simulink model "gm_UZ_EnDat_be4_segregation"  (R2023b)
settings: Solver=FixedStepAuto  StartTime=0  StopTime=0.000505  RelTol=1e-3
model workspace (MAT data in the model file):
  Select = 0
libraries: hdlsllib x74, simulink x21, hdlmdlgenlib x4, simulink_extras x1
(part 5 of 5)

== system gm_UZ_EnDat_be4_segregation/UZ_ENDAT/ManualDeserializere/ramwatcher/Increment Stored Integer ==
  u : Inport  OutDataTypeStr=fixdt(0,16,0,'DataTypeOverride', 'Off')  SampleTime=1e-08
  FixPt Constant : Constant  DisableCoverage=on  OutDataTypeStr=Inherit: Inherit via back propagation  SampleTime=-1
  FixPt Data Type Duplicate : DataTypeDuplicate  DisableCoverage=on  NumInputPorts=3
  FixPt Gateway In : DataTypeConversion  DisableCoverage=on  ConvertRealWorld=Stored Integer (SI)  SaturateOnIntegerOverflow=off  RndMeth=Floor
  FixPt Sum1 : Sum  OutDataTypeStr=Inherit: Inherit via back propagation  InputSameDT=on  LockScale=on
  sigspec : SignalSpecification  OutDataTypeStr=uint16  Dimensions=1
  y : Outport  SampleTime=1e-08  InitialOutput=0
  wires:
  u/1 -> FixPt Sum1/1, FixPt Data Type Duplicate/2
  FixPt Constant/1 -> sigspec/1
  FixPt Gateway In/1 -> FixPt Sum1/2, FixPt Data Type Duplicate/3
  FixPt Sum1/1 -> FixPt Data Type Duplicate/1, y/1
  sigspec/1 -> FixPt Gateway In/1

== system gm_UZ_EnDat_be4_segregation/UZ_ENDAT/ManualSerialize/CLKCNTER_RECIEVE/Positional_Counter ==
  valueout : Inport  OutDataTypeStr=uint32  PortDimensions=1  SampleTime=1e-08
  Trigger : Inport  Port=2  OutDataTypeStr=boolean  SampleTime=1e-08
  Increment Stored Integer : Subsystem  mask(Stored Integer Value Increment){}
      mask help: Simulink:masks:StoredIntegerValueIncrement_MD
      mask Display: disp('Q++')
  Increment Stored Integer_out1bypassMux : MultiPortSwitch  DataPortOrder=Zero-based contiguous  Inputs=2  zeroidx=on  OutDataTypeStr=uint32  SampleTime=1e-08  SaturateOnIntegerOverflow=off  InputSameDT=off
  Trigger_delay : Delay  DelayLength=double(1)  InitialCondition=0
  Trigger_delayed_inverted_and_Trigger : Logic  AllPortsSameDT=off  OutDataTypeStr=boolean  SampleTime=1e-08
  not_Trigger_delayed : Logic  Operator=NOT  Inputs=1  AllPortsSameDT=off  OutDataTypeStr=boolean  SampleTime=1e-08
  out0_bypass : UnitDelay  InitialCondition="fi(0,0,32,0,\"hex\",\"00000000\")"  SampleTime=1e-08
  divider : Outport  SampleTime=1e-08  InitialOutput=0
  wires:
  Trigger/1 -> Trigger_delayed_inverted_and_Trigger/2, Trigger_delay/1
  valueout/1 -> Increment Stored Integer/1(u)
  Increment Stored Integer_out1bypassMux/1 -> divider/1, out0_bypass/1
  Trigger_delay/1 -> not_Trigger_delayed/1
  not_Trigger_delayed/1 -> Trigger_delayed_inverted_and_Trigger/1
  Trigger_delayed_inverted_and_Trigger/1 -> Increment Stored Integer_out1bypassMux/1
  out0_bypass/1 -> Increment Stored Integer_out1bypassMux/2
  Increment Stored Integer/1(y) -> Increment Stored Integer_out1bypassMux/3

== system gm_UZ_EnDat_be4_segregation/UZ_ENDAT/ManualSerialize/CLKCNTER_RECIEVE/SetZero32 ==
  valin : Inport  OutDataTypeStr=uint32  PortDimensions=1  SampleTime=1e-08
  setzero : Inport  Port=2  OutDataTypeStr=boolean  PortDimensions=1  SampleTime=1e-08
  Trigger : Inport  Port=3  OutDataTypeStr=boolean  SampleTime=1e-08
  Constant1 : Constant  OutDataTypeStr=fixdt(0, 1, 0)  SampleTime=1e-08
  Constant2 : Constant  Value=0  OutDataTypeStr=fixdt(0, 1, 0)  SampleTime=1e-08
  Index Vector1 : MultiPortSwitch  DataPortOrder=Zero-based contiguous  Inputs=2  DiagnosticForDefault=None  zeroidx=on  OutDataTypeStr=fixdt(0, 1, 0)  SampleTime=1e-08  SaturateOnIntegerOverflow=off  InputSameDT=off
  Product : Product  Inputs=**  OutDataTypeStr=uint32  SaturateOnIntegerOverflow=on  SampleTime=1e-08
  Product_out1bypassMux : MultiPortSwitch  DataPortOrder=Zero-based contiguous  Inputs=2  zeroidx=on  OutDataTypeStr=uint32  SampleTime=1e-08  SaturateOnIntegerOverflow=off  InputSameDT=off
  Trigger_delay : Delay  DelayLength=double(1)  InitialCondition=0
  Trigger_delay_Initial_Val : Constant  OutDataTypeStr=boolean  SampleTime=1e-08
  Trigger_delay_ctrl_const : Constant  OutDataTypeStr=boolean  SampleTime=1e-08
  Trigger_delay_ctrl_delay : Delay  DelayLength=double(1)  InitialCondition=0
  Trigger_delay_switch : Switch  Criteria=u2 ~= 0  Threshold=double(0)  OutDataTypeStr=boolean  SampleTime=1e-08  SaturateOnIntegerOverflow=off  InputSameDT=off
  Trigger_delayed_inverted_and_Trigger : Logic  AllPortsSameDT=off  OutDataTypeStr=boolean  SampleTime=1e-08
  delayMatch{,1..5} (6 alike) : Delay  DelayLength=double(2)  InitialCondition=0
  not_Trigger_delayed : Logic  Operator=NOT  Inputs=1  AllPortsSameDT=off  OutDataTypeStr=boolean  SampleTime=1e-08
  out0_bypass : UnitDelay  InitialCondition=double(0)  SampleTime=1e-08
  out0_bypass_Initial_Val : Constant  OutDataTypeStr=uint32  SampleTime=1e-08
  out0_bypass_ctrl_const : Constant  OutDataTypeStr=boolean  SampleTime=1e-08
  out0_bypass_ctrl_delay : Delay  DelayLength=double(1)  InitialCondition=0
  out0_bypass_switch : Switch  Criteria=u2 ~= 0  Threshold=double(0)  OutDataTypeStr=uint32  SampleTime=1e-08  SaturateOnIntegerOverflow=off  InputSameDT=off
  valueout : Outport  SampleTime=1e-08  InitialOutput=0  VectorParamsAs1DForOutWhenUnconnected=off
  wires:
  Trigger/1 -> Trigger_delayed_inverted_and_Trigger/2, Trigger_delay/1
  valin/1 -> Product/2
  setzero/1 -> Index Vector1/1
  Trigger_delay_switch/1 -> not_Trigger_delayed/1
  not_Trigger_delayed/1 -> Trigger_delayed_inverted_and_Trigger/1
  Trigger_delay/1 -> Trigger_delay_switch/1
  delayMatch1/1 -> Trigger_delay_switch/3
  delayMatch/1 -> Trigger_delay_switch/2
  Index Vector1/1 -> Product/1
  delayMatch2/1 -> Index Vector1/2
  delayMatch3/1 -> Index Vector1/3
  Trigger_delay_ctrl_delay/1 -> delayMatch/1
  Trigger_delay_Initial_Val/1 -> delayMatch1/1
  Constant1/1 -> delayMatch2/1
  Constant2/1 -> delayMatch3/1
  out0_bypass_ctrl_delay/1 -> delayMatch4/1
  out0_bypass_Initial_Val/1 -> delayMatch5/1
  Product_out1bypassMux/1 -> out0_bypass/1, valueout/1
  out0_bypass/1 -> out0_bypass_switch/1
  delayMatch4/1 -> out0_bypass_switch/2
  delayMatch5/1 -> out0_bypass_switch/3
  Trigger_delayed_inverted_and_Trigger/1 -> Product_out1bypassMux/1
  Product/1 -> Product_out1bypassMux/3
  out0_bypass_switch/1 -> Product_out1bypassMux/2
  out0_bypass_ctrl_const/1 -> out0_bypass_ctrl_delay/1
  Trigger_delay_ctrl_const/1 -> Trigger_delay_ctrl_delay/1

== system gm_UZ_EnDat_be4_segregation/UZ_ENDAT/ManualSerialize/Storage16/Compare To Zero ==
  u : Inport  OutDataTypeStr=fixdt(0,64,0,'DataTypeOverride', 'Off')  SampleTime=1e-08
  Compare : RelationalOperator  Operator===  OutDataTypeStr=boolean
  Constant : Constant  DisableCoverage=on  Value=0  OutDataTypeStr=Inherit: Inherit via back propagation  SampleTime=-1  PreserveConstantTs=on
  y : Outport  SampleTime=1e-08
  wires:
  u/1 -> Compare/1
  Compare/1 -> y/1
  Constant/1 -> Compare/2

== system gm_UZ_EnDat_be4_segregation/UZ_ENDAT/Subsystem/CLKCNTERBOOTUP/Positional_Counter ==
  valueout : Inport  OutDataTypeStr=fixdt(0, 64, 0)  PortDimensions=1  SampleTime=1e-08
  Trigger : Inport  Port=2  OutDataTypeStr=boolean  SampleTime=1e-08
  Increment Stored Integer : Subsystem  mask(Stored Integer Value Increment){}
      mask help: Simulink:masks:StoredIntegerValueIncrement_MD
      mask Display: disp('Q++')
  Increment Stored Integer_out1bypassMux : MultiPortSwitch  DataPortOrder=Zero-based contiguous  Inputs=2  zeroidx=on  OutDataTypeStr=fixdt(0, 64, 0)  SampleTime=1e-08  SaturateOnIntegerOverflow=off  InputSameDT=off
  Trigger_delay : Delay  DelayLength=double(1)  InitialCondition=0
  Trigger_delayed_inverted_and_Trigger : Logic  AllPortsSameDT=off  OutDataTypeStr=boolean  SampleTime=1e-08
  not_Trigger_delayed : Logic  Operator=NOT  Inputs=1  AllPortsSameDT=off  OutDataTypeStr=boolean  SampleTime=1e-08
  out0_bypass : UnitDelay  InitialCondition="fi(0,0,64,0,\"hex\",\"0000000000000000\")"  SampleTime=1e-08
  divider : Outport  SampleTime=1e-08  InitialOutput=0
  wires:
  Trigger/1 -> Trigger_delayed_inverted_and_Trigger/2, Trigger_delay/1
  valueout/1 -> Increment Stored Integer/1(u)
  Increment Stored Integer_out1bypassMux/1 -> divider/1, out0_bypass/1
  Trigger_delay/1 -> not_Trigger_delayed/1
  not_Trigger_delayed/1 -> Trigger_delayed_inverted_and_Trigger/1
  Trigger_delayed_inverted_and_Trigger/1 -> Increment Stored Integer_out1bypassMux/1
  out0_bypass/1 -> Increment Stored Integer_out1bypassMux/2
  Increment Stored Integer/1(y) -> Increment Stored Integer_out1bypassMux/3

== system gm_UZ_EnDat_be4_segregation/UZ_ENDAT/Subsystem/CLKCNTERBOOTUP/SetZero64 ==
  valin : Inport  OutDataTypeStr=fixdt(0, 64, 0)  PortDimensions=1  SampleTime=1e-08
  setzero : Inport  Port=2  OutDataTypeStr=boolean  PortDimensions=1  SampleTime=1e-08
  Trigger : Inport  Port=3  OutDataTypeStr=boolean  SampleTime=1e-08
  Constant1 : Constant  OutDataTypeStr=fixdt(0, 1, 0)  SampleTime=1e-08
  Constant2 : Constant  Value=0  OutDataTypeStr=fixdt(0, 1, 0)  SampleTime=1e-08
  Index Vector1 : MultiPortSwitch  DataPortOrder=Zero-based contiguous  Inputs=2  DiagnosticForDefault=None  zeroidx=on  OutDataTypeStr=fixdt(0, 1, 0)  SampleTime=1e-08  SaturateOnIntegerOverflow=off  InputSameDT=off
  Product : Product  Inputs=**  OutDataTypeStr=fixdt(0, 64, 0)  SaturateOnIntegerOverflow=on  SampleTime=1e-08
  Product_out1bypassMux : MultiPortSwitch  DataPortOrder=Zero-based contiguous  Inputs=2  zeroidx=on  OutDataTypeStr=fixdt(0, 64, 0)  SampleTime=1e-08  SaturateOnIntegerOverflow=off  InputSameDT=off
  Trigger_delay : Delay  DelayLength=double(1)  InitialCondition=0
  Trigger_delay_Initial_Val : Constant  OutDataTypeStr=boolean  SampleTime=1e-08
  Trigger_delay_ctrl_const : Constant  OutDataTypeStr=boolean  SampleTime=1e-08
  Trigger_delay_ctrl_delay : Delay  DelayLength=double(1)  InitialCondition=0
  Trigger_delay_switch : Switch  Criteria=u2 ~= 0  Threshold=double(0)  OutDataTypeStr=boolean  SampleTime=1e-08  SaturateOnIntegerOverflow=off  InputSameDT=off
  Trigger_delayed_inverted_and_Trigger : Logic  AllPortsSameDT=off  OutDataTypeStr=boolean  SampleTime=1e-08
  not_Trigger_delayed : Logic  Operator=NOT  Inputs=1  AllPortsSameDT=off  OutDataTypeStr=boolean  SampleTime=1e-08
  out0_bypass : UnitDelay  InitialCondition=double(0)  SampleTime=1e-08
  out0_bypass_Initial_Val : Constant  Value="fi(0,0,64,0,\"hex\",\"0000000000000001\")"  OutDataTypeStr=fixdt(0, 64, 0)  SampleTime=1e-08
  out0_bypass_ctrl_const : Constant  OutDataTypeStr=boolean  SampleTime=1e-08
  out0_bypass_ctrl_delay : Delay  DelayLength=double(1)  InitialCondition=0
  out0_bypass_switch : Switch  Criteria=u2 ~= 0  Threshold=double(0)  OutDataTypeStr=fixdt(0, 64, 0)  SampleTime=1e-08  SaturateOnIntegerOverflow=off  InputSameDT=off
  valueout : Outport  SampleTime=1e-08  InitialOutput=0  VectorParamsAs1DForOutWhenUnconnected=off
  wires:
  Trigger/1 -> Trigger_delayed_inverted_and_Trigger/2, Trigger_delay/1
  valin/1 -> Product/2
  setzero/1 -> Index Vector1/1
  Product_out1bypassMux/1 -> valueout/1, out0_bypass/1
  Trigger_delay_switch/1 -> not_Trigger_delayed/1
  not_Trigger_delayed/1 -> Trigger_delayed_inverted_and_Trigger/1
  Trigger_delay/1 -> Trigger_delay_switch/1
  Trigger_delay_Initial_Val/1 -> Trigger_delay_switch/3
  Trigger_delay_ctrl_delay/1 -> Trigger_delay_switch/2
  Index Vector1/1 -> Product/1
  Constant1/1 -> Index Vector1/2
  Constant2/1 -> Index Vector1/3
  out0_bypass/1 -> out0_bypass_switch/1
  out0_bypass_ctrl_delay/1 -> out0_bypass_switch/2
  out0_bypass_Initial_Val/1 -> out0_bypass_switch/3
  Trigger_delayed_inverted_and_Trigger/1 -> Product_out1bypassMux/1
  Product/1 -> Product_out1bypassMux/3
  out0_bypass_switch/1 -> Product_out1bypassMux/2
  out0_bypass_ctrl_const/1 -> out0_bypass_ctrl_delay/1
  Trigger_delay_ctrl_const/1 -> Trigger_delay_ctrl_delay/1

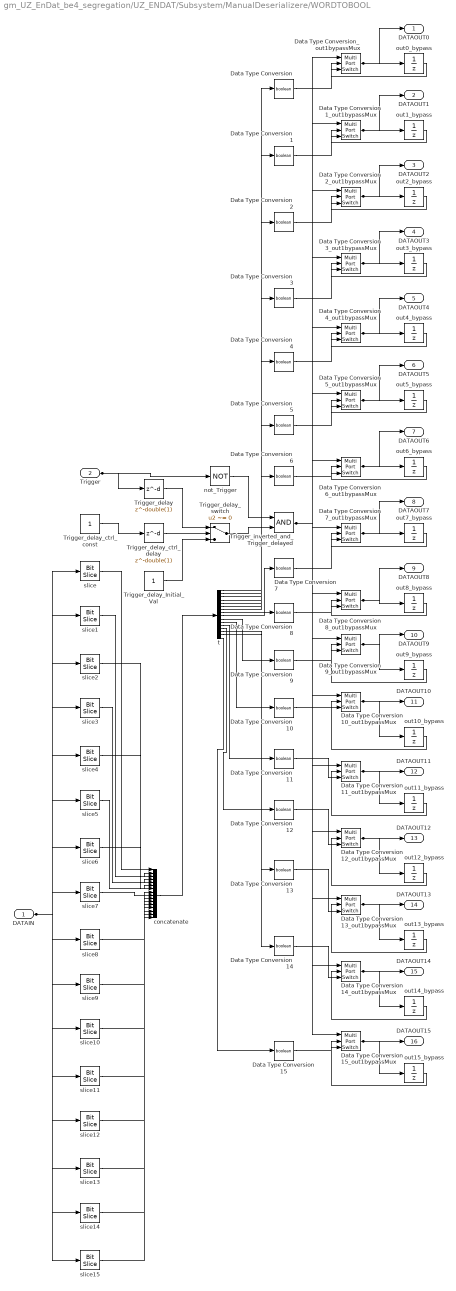
== system gm_UZ_EnDat_be4_segregation/UZ_ENDAT/Subsystem/ManualDeserializere/WORDTOBOOL ==
  DATAIN : Inport  OutDataTypeStr=uint16  PortDimensions=1  SampleTime=1e-08
  Trigger : Inport  Port=2  OutDataTypeStr=boolean  SampleTime=1e-08
  Data Type Conversion{,1..15} (16 alike) : DataTypeConversion  OutDataTypeStr=boolean  SampleTime=1e-08  SaturateOnIntegerOverflow=off  RndMeth=Floor
  Data Type Conversion10_out1bypassMux : MultiPortSwitch  DataPortOrder=Zero-based contiguous  Inputs=2  zeroidx=on  SampleTime=1e-08  SaturateOnIntegerOverflow=off  InputSameDT=off
  Data Type Conversion11_out1bypassMux : MultiPortSwitch  DataPortOrder=Zero-based contiguous  Inputs=2  zeroidx=on  SampleTime=1e-08  SaturateOnIntegerOverflow=off  InputSameDT=off
  Data Type Conversion12_out1bypassMux : MultiPortSwitch  DataPortOrder=Zero-based contiguous  Inputs=2  zeroidx=on  SampleTime=1e-08  SaturateOnIntegerOverflow=off  InputSameDT=off
  Data Type Conversion13_out1bypassMux : MultiPortSwitch  DataPortOrder=Zero-based contiguous  Inputs=2  zeroidx=on  SampleTime=1e-08  SaturateOnIntegerOverflow=off  InputSameDT=off
  Data Type Conversion14_out1bypassMux : MultiPortSwitch  DataPortOrder=Zero-based contiguous  Inputs=2  zeroidx=on  SampleTime=1e-08  SaturateOnIntegerOverflow=off  InputSameDT=off
  Data Type Conversion15_out1bypassMux : MultiPortSwitch  DataPortOrder=Zero-based contiguous  Inputs=2  zeroidx=on  SampleTime=1e-08  SaturateOnIntegerOverflow=off  InputSameDT=off
  Data Type Conversion1_out1bypassMux : MultiPortSwitch  DataPortOrder=Zero-based contiguous  Inputs=2  zeroidx=on  SampleTime=1e-08  SaturateOnIntegerOverflow=off  InputSameDT=off
  Data Type Conversion2_out1bypassMux : MultiPortSwitch  DataPortOrder=Zero-based contiguous  Inputs=2  zeroidx=on  SampleTime=1e-08  SaturateOnIntegerOverflow=off  InputSameDT=off
  Data Type Conversion3_out1bypassMux : MultiPortSwitch  DataPortOrder=Zero-based contiguous  Inputs=2  zeroidx=on  SampleTime=1e-08  SaturateOnIntegerOverflow=off  InputSameDT=off
  Data Type Conversion4_out1bypassMux : MultiPortSwitch  DataPortOrder=Zero-based contiguous  Inputs=2  zeroidx=on  SampleTime=1e-08  SaturateOnIntegerOverflow=off  InputSameDT=off
  Data Type Conversion5_out1bypassMux : MultiPortSwitch  DataPortOrder=Zero-based contiguous  Inputs=2  zeroidx=on  SampleTime=1e-08  SaturateOnIntegerOverflow=off  InputSameDT=off
  Data Type Conversion6_out1bypassMux : MultiPortSwitch  DataPortOrder=Zero-based contiguous  Inputs=2  zeroidx=on  SampleTime=1e-08  SaturateOnIntegerOverflow=off  InputSameDT=off
  Data Type Conversion7_out1bypassMux : MultiPortSwitch  DataPortOrder=Zero-based contiguous  Inputs=2  zeroidx=on  SampleTime=1e-08  SaturateOnIntegerOverflow=off  InputSameDT=off
  Data Type Conversion8_out1bypassMux : MultiPortSwitch  DataPortOrder=Zero-based contiguous  Inputs=2  zeroidx=on  SampleTime=1e-08  SaturateOnIntegerOverflow=off  InputSameDT=off
  Data Type Conversion9_out1bypassMux : MultiPortSwitch  DataPortOrder=Zero-based contiguous  Inputs=2  zeroidx=on  SampleTime=1e-08  SaturateOnIntegerOverflow=off  InputSameDT=off
  Data Type Conversion_out1bypassMux : MultiPortSwitch  DataPortOrder=Zero-based contiguous  Inputs=2  zeroidx=on  SampleTime=1e-08  SaturateOnIntegerOverflow=off  InputSameDT=off
  Trigger_delay : Delay  DelayLength=double(1)  InitialCondition=0
  Trigger_delay_Initial_Val : Constant  OutDataTypeStr=boolean  SampleTime=1e-08
  Trigger_delay_ctrl_const : Constant  OutDataTypeStr=boolean  SampleTime=1e-08
  Trigger_delay_ctrl_delay : Delay  DelayLength=double(1)  InitialCondition=0
  Trigger_delay_switch : Switch  Criteria=u2 ~= 0  Threshold=double(0)  OutDataTypeStr=boolean  SampleTime=1e-08  SaturateOnIntegerOverflow=off  InputSameDT=off
  Trigger_inverted_and_Trigger_delayed : Logic  AllPortsSameDT=off  OutDataTypeStr=boolean  SampleTime=1e-08
  concatenate : Concatenate  NumInputs=16  Mode=Multidimensional array  ConcatenateDimension=2
  not_Trigger : Logic  Operator=NOT  Inputs=1  AllPortsSameDT=off  OutDataTypeStr=boolean  SampleTime=1e-08
  out0_bypass : UnitDelay  SampleTime=1e-08
  out10_bypass : UnitDelay  SampleTime=1e-08
  out11_bypass : UnitDelay  SampleTime=1e-08
  out12_bypass : UnitDelay  SampleTime=1e-08
  out13_bypass : UnitDelay  SampleTime=1e-08
  out14_bypass : UnitDelay  SampleTime=1e-08
  out15_bypass : UnitDelay  SampleTime=1e-08
  out1_bypass : UnitDelay  SampleTime=1e-08
  out2_bypass : UnitDelay  SampleTime=1e-08
  out3_bypass : UnitDelay  SampleTime=1e-08
  out4_bypass : UnitDelay  SampleTime=1e-08
  out5_bypass : UnitDelay  SampleTime=1e-08
  out6_bypass : UnitDelay  SampleTime=1e-08
  out7_bypass : UnitDelay  SampleTime=1e-08
  out8_bypass : UnitDelay  SampleTime=1e-08
  out9_bypass : UnitDelay  SampleTime=1e-08
  slice : hdlsllib/Logic and Bit Operations/Bit Slice  lidx=double(0)  ridx=double(0)
  slice1 : hdlsllib/Logic and Bit Operations/Bit Slice  lidx=double(1)  ridx=double(1)
  slice10 : hdlsllib/Logic and Bit Operations/Bit Slice  lidx=double(10)  ridx=double(10)
  slice11 : hdlsllib/Logic and Bit Operations/Bit Slice  lidx=double(11)  ridx=double(11)
  slice12 : hdlsllib/Logic and Bit Operations/Bit Slice  lidx=double(12)  ridx=double(12)
  slice13 : hdlsllib/Logic and Bit Operations/Bit Slice  lidx=double(13)  ridx=double(13)
  slice14 : hdlsllib/Logic and Bit Operations/Bit Slice  lidx=double(14)  ridx=double(14)
  slice15 : hdlsllib/Logic and Bit Operations/Bit Slice  lidx=double(15)  ridx=double(15)
  slice2 : hdlsllib/Logic and Bit Operations/Bit Slice  lidx=double(2)  ridx=double(2)
  slice3 : hdlsllib/Logic and Bit Operations/Bit Slice  lidx=double(3)  ridx=double(3)
  slice4 : hdlsllib/Logic and Bit Operations/Bit Slice  lidx=double(4)  ridx=double(4)
  slice5 : hdlsllib/Logic and Bit Operations/Bit Slice  lidx=double(5)  ridx=double(5)
  slice6 : hdlsllib/Logic and Bit Operations/Bit Slice  lidx=double(6)  ridx=double(6)
  slice7 : hdlsllib/Logic and Bit Operations/Bit Slice  lidx=double(7)  ridx=double(7)
  slice8 : hdlsllib/Logic and Bit Operations/Bit Slice  lidx=double(8)  ridx=double(8)
  slice9 : hdlsllib/Logic and Bit Operations/Bit Slice  lidx=double(9)  ridx=double(9)
  t : Demux  Outputs=16
  DATAOUT0 : Outport  SampleTime=1e-08  InitialOutput=0
  DATAOUT1 : Outport  Port=2  SampleTime=1e-08  InitialOutput=0
  DATAOUT2 : Outport  Port=3  SampleTime=1e-08  InitialOutput=0
  DATAOUT3 : Outport  Port=4  SampleTime=1e-08  InitialOutput=0
  DATAOUT4 : Outport  Port=5  SampleTime=1e-08  InitialOutput=0
  DATAOUT5 : Outport  Port=6  SampleTime=1e-08  InitialOutput=0
  DATAOUT6 : Outport  Port=7  SampleTime=1e-08  InitialOutput=0
  DATAOUT7 : Outport  Port=8  SampleTime=1e-08  InitialOutput=0
  DATAOUT8 : Outport  Port=9  SampleTime=1e-08  InitialOutput=0
  DATAOUT9 : Outport  Port=10  SampleTime=1e-08  InitialOutput=0
  DATAOUT10 : Outport  Port=11  SampleTime=1e-08  InitialOutput=0
  DATAOUT11 : Outport  Port=12  SampleTime=1e-08  InitialOutput=0
  DATAOUT12 : Outport  Port=13  SampleTime=1e-08  InitialOutput=0
  DATAOUT13 : Outport  Port=14  SampleTime=1e-08  InitialOutput=0
  DATAOUT14 : Outport  Port=15  SampleTime=1e-08  InitialOutput=0
  DATAOUT15 : Outport  Port=16  SampleTime=1e-08  InitialOutput=0
  wires:
  Trigger/1 -> not_Trigger/1, Trigger_delay/1
  DATAIN/1 -> slice15/1, slice14/1, slice13/1, slice12/1, slice11/1, slice10/1, slice9/1, slice8/1, slice7/1, slice6/1, slice5/1, slice4/1, slice3/1, slice2/1, slice1/1, slice/1
  Data Type Conversion_out1bypassMux/1 -> DATAOUT0/1, out0_bypass/1
  Data Type Conversion1_out1bypassMux/1 -> DATAOUT1/1, out1_bypass/1
  Data Type Conversion2_out1bypassMux/1 -> DATAOUT2/1, out2_bypass/1
  Data Type Conversion3_out1bypassMux/1 -> DATAOUT3/1, out3_bypass/1
  Data Type Conversion4_out1bypassMux/1 -> DATAOUT4/1, out4_bypass/1
  Data Type Conversion5_out1bypassMux/1 -> DATAOUT5/1, out5_bypass/1
  Data Type Conversion6_out1bypassMux/1 -> DATAOUT6/1, out6_bypass/1
  Data Type Conversion7_out1bypassMux/1 -> DATAOUT7/1, out7_bypass/1
  Data Type Conversion8_out1bypassMux/1 -> DATAOUT8/1, out8_bypass/1
  Data Type Conversion9_out1bypassMux/1 -> DATAOUT9/1, out9_bypass/1
  Data Type Conversion10_out1bypassMux/1 -> DATAOUT10/1, out10_bypass/1
  Data Type Conversion11_out1bypassMux/1 -> DATAOUT11/1, out11_bypass/1
  Data Type Conversion12_out1bypassMux/1 -> DATAOUT12/1, out12_bypass/1
  Data Type Conversion13_out1bypassMux/1 -> DATAOUT13/1, out13_bypass/1
  Data Type Conversion14_out1bypassMux/1 -> DATAOUT14/1, out14_bypass/1
  Data Type Conversion15_out1bypassMux/1 -> DATAOUT15/1, out15_bypass/1
  Trigger_delay_switch/1 -> Trigger_inverted_and_Trigger_delayed/2
  not_Trigger/1 -> Trigger_inverted_and_Trigger_delayed/1
  Trigger_inverted_and_Trigger_delayed/1 -> Data Type Conversion_out1bypassMux/1, Data Type Conversion1_out1bypassMux/1, Data Type Conversion2_out1bypassMux/1, Data Type Conversion3_out1bypassMux/1, Data Type Conversion4_out1bypassMux/1, Data Type Conversion5_out1bypassMux/1, Data Type Conversion6_out1bypassMux/1, Data Type Conversion7_out1bypassMux/1, Data Type Conversion8_out1bypassMux/1, Data Type Conversion9_out1bypassMux/1, Data Type Conversion10_out1bypassMux/1, Data Type Conversion11_out1bypassMux/1, Data Type Conversion12_out1bypassMux/1, Data Type Conversion13_out1bypassMux/1, Data Type Conversion14_out1bypassMux/1, Data Type Conversion15_out1bypassMux/1
  Trigger_delay/1 -> Trigger_delay_switch/1
  Trigger_delay_Initial_Val/1 -> Trigger_delay_switch/3
  Trigger_delay_ctrl_const/1 -> Trigger_delay_ctrl_delay/1
  Trigger_delay_ctrl_delay/1 -> Trigger_delay_switch/2
  concatenate/1 -> t/1
  t/1 -> Data Type Conversion/1
  t/2 -> Data Type Conversion1/1
  t/3 -> Data Type Conversion2/1
  t/4 -> Data Type Conversion3/1
  t/5 -> Data Type Conversion4/1
  t/6 -> Data Type Conversion5/1
  t/7 -> Data Type Conversion6/1
  t/8 -> Data Type Conversion7/1
  t/9 -> Data Type Conversion8/1
  t/10 -> Data Type Conversion9/1
  t/11 -> Data Type Conversion10/1
  t/12 -> Data Type Conversion11/1
  t/13 -> Data Type Conversion12/1
  t/14 -> Data Type Conversion13/1
  t/15 -> Data Type Conversion14/1
  t/16 -> Data Type Conversion15/1
  slice/1 -> concatenate/1
  slice1/1 -> concatenate/2
  slice2/1 -> concatenate/3
  slice3/1 -> concatenate/4
  slice4/1 -> concatenate/5
  slice5/1 -> concatenate/6
  slice6/1 -> concatenate/7
  slice7/1 -> concatenate/8
  slice8/1 -> concatenate/9
  slice9/1 -> concatenate/10
  slice10/1 -> concatenate/11
  slice11/1 -> concatenate/12
  slice12/1 -> concatenate/13
  slice13/1 -> concatenate/14
  slice14/1 -> concatenate/15
  slice15/1 -> concatenate/16
  out0_bypass/1 -> Data Type Conversion_out1bypassMux/2
  Data Type Conversion/1 -> Data Type Conversion_out1bypassMux/3
  out1_bypass/1 -> Data Type Conversion1_out1bypassMux/2
  Data Type Conversion1/1 -> Data Type Conversion1_out1bypassMux/3
  out2_bypass/1 -> Data Type Conversion2_out1bypassMux/2
  Data Type Conversion2/1 -> Data Type Conversion2_out1bypassMux/3
  out3_bypass/1 -> Data Type Conversion3_out1bypassMux/2
  Data Type Conversion3/1 -> Data Type Conversion3_out1bypassMux/3
  out4_bypass/1 -> Data Type Conversion4_out1bypassMux/2
  Data Type Conversion4/1 -> Data Type Conversion4_out1bypassMux/3
  out5_bypass/1 -> Data Type Conversion5_out1bypassMux/2
  Data Type Conversion5/1 -> Data Type Conversion5_out1bypassMux/3
  out6_bypass/1 -> Data Type Conversion6_out1bypassMux/2
  Data Type Conversion6/1 -> Data Type Conversion6_out1bypassMux/3
  out7_bypass/1 -> Data Type Conversion7_out1bypassMux/2
  Data Type Conversion7/1 -> Data Type Conversion7_out1bypassMux/3
  out8_bypass/1 -> Data Type Conversion8_out1bypassMux/2
  Data Type Conversion8/1 -> Data Type Conversion8_out1bypassMux/3
  out9_bypass/1 -> Data Type Conversion9_out1bypassMux/2
  Data Type Conversion9/1 -> Data Type Conversion9_out1bypassMux/3
  out10_bypass/1 -> Data Type Conversion10_out1bypassMux/2
  Data Type Conversion10/1 -> Data Type Conversion10_out1bypassMux/3
  out11_bypass/1 -> Data Type Conversion11_out1bypassMux/2
  Data Type Conversion11/1 -> Data Type Conversion11_out1bypassMux/3
  out12_bypass/1 -> Data Type Conversion12_out1bypassMux/2
  Data Type Conversion12/1 -> Data Type Conversion12_out1bypassMux/3
  out13_bypass/1 -> Data Type Conversion13_out1bypassMux/2
  Data Type Conversion13/1 -> Data Type Conversion13_out1bypassMux/3
  out14_bypass/1 -> Data Type Conversion14_out1bypassMux/2
  Data Type Conversion14/1 -> Data Type Conversion14_out1bypassMux/3
  out15_bypass/1 -> Data Type Conversion15_out1bypassMux/2
  Data Type Conversion15/1 -> Data Type Conversion15_out1bypassMux/3

== system gm_UZ_EnDat_be4_segregation/UZ_ENDAT/Subsystem/ManualDeserializere/ramwatcher ==
  In1 : Inport  OutMin=0  OutMax=32000  OutDataTypeStr=uint16  PortDimensions=1  SampleTime=1e-08  LockScale=on
  In2 : Inport  Port=2  OutMin=0  OutMax=1  OutDataTypeStr=fixdt(0, 1, 0)  PortDimensions=1  SampleTime=1e-08  LockScale=on
  Trigger : Inport  Port=3  OutDataTypeStr=boolean  SampleTime=1e-08
  Increment Stored Integer : Subsystem  mask(Stored Integer Value Increment){}
      mask help: Simulink:masks:StoredIntegerValueIncrement_MD
      mask Display: disp('Q++')
  Product : Product  Inputs=**  OutDataTypeStr=uint16  SampleTime=1e-08
  Product_out1bypassMux : MultiPortSwitch  DataPortOrder=Zero-based contiguous  Inputs=2  zeroidx=on  OutDataTypeStr=uint16  SampleTime=1e-08  SaturateOnIntegerOverflow=off  InputSameDT=off
  Trigger_delay : Delay  DelayLength=double(1)  InitialCondition=0
  Trigger_delayed_inverted_and_Trigger : Logic  AllPortsSameDT=off  OutDataTypeStr=boolean  SampleTime=1e-08
  not_Trigger_delayed : Logic  Operator=NOT  Inputs=1  AllPortsSameDT=off  OutDataTypeStr=boolean  SampleTime=1e-08
  out0_bypass : UnitDelay  InitialCondition="fi(0,0,16,0,\"hex\",\"0000\")"  SampleTime=1e-08
  SEL : Outport  SampleTime=1e-08  InitialOutput=0
  wires:
  Product/1 -> Product_out1bypassMux/3
  out0_bypass/1 -> Product_out1bypassMux/2
  Trigger_delayed_inverted_and_Trigger/1 -> Product_out1bypassMux/1
  Increment Stored Integer/1(y) -> Product/1
  not_Trigger_delayed/1 -> Trigger_delayed_inverted_and_Trigger/1
  Trigger_delay/1 -> not_Trigger_delayed/1
  Product_out1bypassMux/1 -> out0_bypass/1, SEL/1
  In2/1 -> Product/2
  In1/1 -> Increment Stored Integer/1(u)
  Trigger/1 -> Trigger_delay/1, Trigger_delayed_inverted_and_Trigger/2

== system gm_UZ_EnDat_be4_segregation/UZ_ENDAT/5timestorage/Triggered Subsystem/Counter Limited/Increment Real World ==
  u : Inport  OutDataTypeStr=fixdt(0,8,0,'DataTypeOverride', 'Off')  SampleTime=1e-08
  FixPt Constant : Constant  OutDataTypeStr=uint8  SampleTime=1e-08
  FixPt Data Type Duplicate : DataTypeDuplicate  DisableCoverage=on  NumInputPorts=3
  FixPt Sum1 : Sum  OutDataTypeStr=uint8  AccumDataTypeStr=uint8  SampleTime=1e-08
  delayMatch : Delay  DelayLength=double(2)  InitialCondition=0
  delayMatch1 : Delay  DelayLength=double(2)  InitialCondition=0
  y : Outport  SampleTime=1e-08  InitialOutput=0
  wires:
  u/1 -> FixPt Sum1/1, FixPt Data Type Duplicate/2
  delayMatch/1 -> FixPt Sum1/2
  FixPt Sum1/1 -> FixPt Data Type Duplicate/1, y/1
  delayMatch1/1 -> FixPt Data Type Duplicate/3
  FixPt Constant/1 -> delayMatch1/1, delayMatch/1

== system gm_UZ_EnDat_be4_segregation/UZ_ENDAT/5timestorage/Triggered Subsystem/Counter Limited/Output ==
  in0 : Inport  OutDataTypeStr=fixdt(0,8,0,'DataTypeOverride', 'Off')  SampleTime=1e-08
  Trigger_emulated : EnablePort  OutDataTypeStr=boolean
  Output : Delay  DelayLength=double(1)  InitialCondition=0
  out0 : Outport  OutDataTypeStr=fixdt(0,8,0,'DataTypeOverride', 'Off')  SampleTime=1e-08  InitialOutput=0
  wires:
  Output/1 -> out0/1
  in0/1 -> Output/1

== system gm_UZ_EnDat_be4_segregation/UZ_ENDAT/5timestorage/Triggered Subsystem/Counter Limited/Wrap To Zero ==
  note: U(k)
  U : Inport  OutDataTypeStr=fixdt(0,8,0,'DataTypeOverride', 'Off')  SampleTime=1e-08
  Constant : Constant  Value=0  OutDataTypeStr=uint8  SampleTime=1e-08
  FixPt Data Type Duplicate1 : DataTypeDuplicate  DisableCoverage=on  NumInputPorts=3
  FixPt Switch : Switch  Criteria=u2 > Threshold  Threshold=double(4)  OutDataTypeStr=uint8  SampleTime=1e-08  SaturateOnIntegerOverflow=off  InputSameDT=off
  delayMatch : Delay  DelayLength=double(2)  InitialCondition=0
  delayMatch1 : Delay  DelayLength=double(2)  InitialCondition=0
  Y : Outport  SampleTime=1e-08  InitialOutput=0
  wires:
  U/1 -> FixPt Switch/3, FixPt Switch/2, FixPt Data Type Duplicate1/2
  delayMatch/1 -> FixPt Switch/1
  FixPt Switch/1 -> FixPt Data Type Duplicate1/1, Y/1
  delayMatch1/1 -> FixPt Data Type Duplicate1/3
  Constant/1 -> delayMatch1/1, delayMatch/1

== system gm_UZ_EnDat_be4_segregation/UZ_ENDAT/ManualSerialize/CLKCNTER_RECIEVE/Positional_Counter/Increment Stored Integer ==
  u : Inport  OutDataTypeStr=fixdt(0,32,0,'DataTypeOverride', 'Off')  SampleTime=1e-08
  FixPt Constant : Constant  DisableCoverage=on  OutDataTypeStr=Inherit: Inherit via back propagation  SampleTime=-1
  FixPt Data Type Duplicate : DataTypeDuplicate  DisableCoverage=on  NumInputPorts=3
  FixPt Gateway In : DataTypeConversion  DisableCoverage=on  ConvertRealWorld=Stored Integer (SI)  SaturateOnIntegerOverflow=off  RndMeth=Floor
  FixPt Sum1 : Sum  OutDataTypeStr=Inherit: Inherit via back propagation  InputSameDT=on  LockScale=on
  sigspec : SignalSpecification  OutDataTypeStr=uint32  Dimensions=1
  y : Outport  SampleTime=1e-08  InitialOutput=0
  wires:
  u/1 -> FixPt Sum1/1, FixPt Data Type Duplicate/2
  FixPt Constant/1 -> sigspec/1
  FixPt Gateway In/1 -> FixPt Sum1/2, FixPt Data Type Duplicate/3
  FixPt Sum1/1 -> FixPt Data Type Duplicate/1, y/1
  sigspec/1 -> FixPt Gateway In/1

== system gm_UZ_EnDat_be4_segregation/UZ_ENDAT/Subsystem/CLKCNTERBOOTUP/Positional_Counter/Increment Stored Integer ==
  u : Inport  OutDataTypeStr=fixdt(0,64,0,'DataTypeOverride', 'Off')  SampleTime=1e-08
  FixPt Constant : Constant  DisableCoverage=on  OutDataTypeStr=Inherit: Inherit via back propagation  SampleTime=-1
  FixPt Data Type Duplicate : DataTypeDuplicate  DisableCoverage=on  NumInputPorts=3
  FixPt Gateway In : DataTypeConversion  DisableCoverage=on  ConvertRealWorld=Stored Integer (SI)  SaturateOnIntegerOverflow=off  RndMeth=Floor
  FixPt Sum1 : Sum  OutDataTypeStr=Inherit: Inherit via back propagation  InputSameDT=on  LockScale=on
  sigspec : SignalSpecification  OutDataTypeStr=fixdt(0, 64, 0)  Dimensions=1
  y : Outport  SampleTime=1e-08  InitialOutput=0
  wires:
  u/1 -> FixPt Sum1/1, FixPt Data Type Duplicate/2
  FixPt Constant/1 -> sigspec/1
  FixPt Gateway In/1 -> FixPt Sum1/2, FixPt Data Type Duplicate/3
  FixPt Sum1/1 -> FixPt Data Type Duplicate/1, y/1
  sigspec/1 -> FixPt Gateway In/1

== system gm_UZ_EnDat_be4_segregation/UZ_ENDAT/Subsystem/ManualDeserializere/ramwatcher/Increment Stored Integer ==
  u : Inport  OutDataTypeStr=fixdt(0,16,0,'DataTypeOverride', 'Off')  SampleTime=1e-08
  FixPt Constant : Constant  DisableCoverage=on  OutDataTypeStr=Inherit: Inherit via back propagation  SampleTime=-1
  FixPt Data Type Duplicate : DataTypeDuplicate  DisableCoverage=on  NumInputPorts=3
  FixPt Gateway In : DataTypeConversion  DisableCoverage=on  ConvertRealWorld=Stored Integer (SI)  SaturateOnIntegerOverflow=off  RndMeth=Floor
  FixPt Sum1 : Sum  OutDataTypeStr=Inherit: Inherit via back propagation  InputSameDT=on  LockScale=on
  sigspec : SignalSpecification  OutDataTypeStr=uint16  Dimensions=1
  y : Outport  SampleTime=1e-08  InitialOutput=0
  wires:
  sigspec/1 -> FixPt Gateway In/1
  FixPt Sum1/1 -> y/1, FixPt Data Type Duplicate/1
  FixPt Gateway In/1 -> FixPt Data Type Duplicate/3, FixPt Sum1/2
  FixPt Constant/1 -> sigspec/1
  u/1 -> FixPt Data Type Duplicate/2, FixPt Sum1/1
